simulink library "MuteRamper"  (R2022b)
settings: Solver=VariableStepAuto  StartTime=0.0  StopTime=10.0  RelTol=1e-3
libraries: MuteRamperBtc x1
settings Model: Creator=db1045444  LastModifiedBy=db1045444
settings SolverCC: AlgebraicLoopSolver=TrustRegion
settings DebuggingCC: UnconnectedInputMsg=warning  UnconnectedOutputMsg=warning  UnconnectedLineMsg=warning  SFMachineParentedDataDiag=warning
settings ModelReferenceCC: EnableRefExpFcnMdlSchedulingChecks=on
settings RTWCC: DLArmComputeVersion=19.05

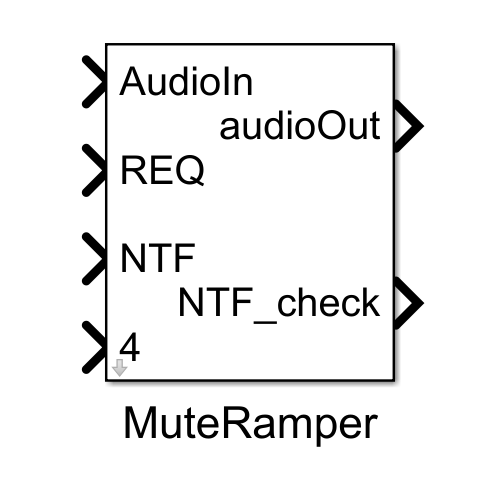
[thumbnail: Simulink's stored preview of the top-level diagram]
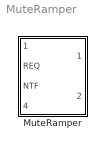
== system MuteRamper ==
  MuteRamper : Subsystem  mask(Bose MuteRamper){MaskFeatureName=Mute, initial_mute_state=1, samplesPerFrame=32}
      mask prompts: MaskFeatureName "InstanceName"; initial_mute_state "Initially muted (logical)"; samplesPerFrame "Samples per Frame"
      mask help: This component is to be used in conjunction with the MuteControl block, which provides runtime control and tuning capabilities via an RTC and the tune variable muteControlRampTime. Multiple instances of this block may be placed within an audio application, and a single MuteControl block has the ability to control all of these rampers simultaneously.
      mask init:
      | blkh = gcbh;
      | % Copy discrete mask parameters into a classdef object
      | InnerLinkConfig = MuteRamperConfig;
      | InnerLinkConfig.InitialMuteState = initial_mute_state;
      | InnerLinkConfig.SamplesPerFrame = samplesPerFrame;
      mask TypeOptions MaskFeatureName: InnerLink/FeatureName

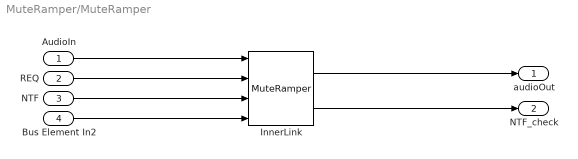
== system MuteRamper/MuteRamper ==
  AudioIn : Inport
  REQ : Inport  Port=2
  NTF : Inport  Port=3
  Bus Element In2 : Inport  Port=4
  InnerLink : MuteRamperBtc/MuteRamper  Config=InnerLinkConfig  FeatureName=Mute
      settings: SourceProductName=Bose Blocklib
  audioOut : Outport
  NTF_check : Outport  Port=2
  wires:
  InnerLink/1 -> audioOut/1
  InnerLink/2 -> NTF_check/1
  AudioIn/1 -> InnerLink/1
  REQ/1 -> InnerLink/2
  NTF/1 -> InnerLink/3
  Bus Element In2/1 -> InnerLink/4
